simulink model "EEG_Acquire_P300_Train_B"  (R2015b)
settings: Solver=FixedStepDiscrete  StartTime=0.0  StopTime=6000  FixedStep=1/250  MaxStep=1/250  RelTol=1e-3
InitFcn:
  | clear global handle
  | 
  | clear global userData
undefined symbols (not defined in the file or in its folder): gcf
settings Model: Creator=ankit  LastModifiedBy=Sun Han
settings SolverCC: AutoInsertRateTranBlk=on  InsertRTBMode=Always
settings DataIOCC: LimitDataPoints=off  SaveFormat=Array  SignalLoggingSaveFormat=ModelDataLogs
settings OptimizationCC: ExpressionDepthLimit=2147483647  InitFltsAndDblsToZero=on
settings DebuggingCC: SaveWithParameterizedLinksMsg=none  UnderspecifiedInitializationDetection=Classic  MergeDetectMultiDrivingBlocksExec=none  SignalResolutionControl=TryResolveAllWithWarning  SolverPrmCheckMsg=warning  MultiTaskDSMMsg=warning  MultiTaskCondExecSysMsg=none  FcnCallInpInsideContextMsg=UseLocalSettings  StateNameClashWarn=warning
settings HardwareCC: ProdBitPerPointer=32  ProdLargestAtomicFloat=None  ProdIntDivRoundTo=Undefined  ProdEndianess=Unspecified  ProdWordSize=32  ProdHWDeviceType=32-bit Generic
settings GRTTargetCC: TargetFcnLib=ansi_tfl_tmw.mat  GeneratePreprocessorConditionals=Disable all  CombineOutputUpdateFcns=off  GRTInterface=on
settings ConfigComp: CovModelRefEnable=Off  CovSFcnEnable=off

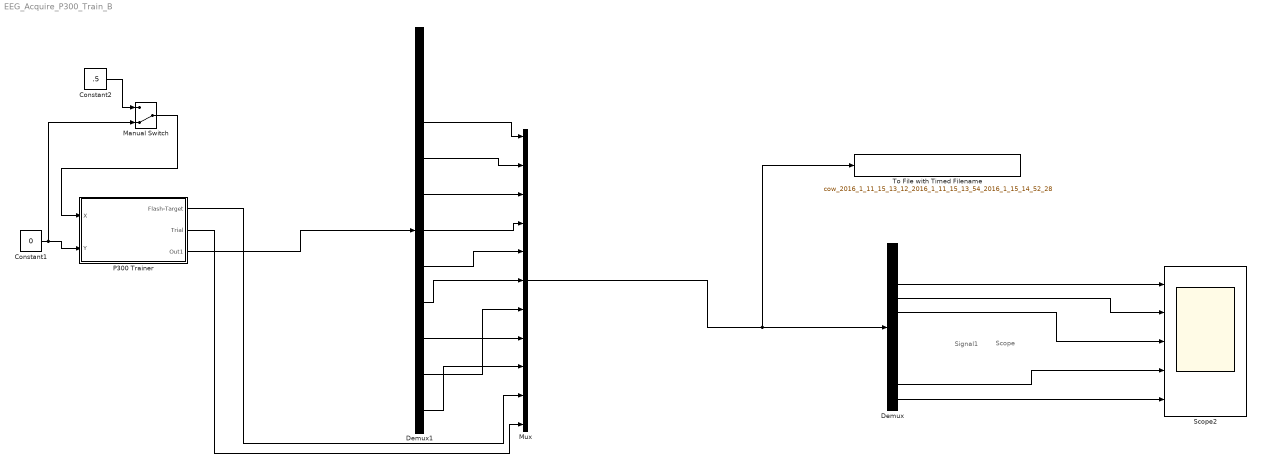
== system EEG_Acquire_P300_Train_B ==
  note: Scope
  note: Signal1
  Constant1 : Constant  Value=0
  Constant2 : Constant  Value=.5
  Demux : Demux  Outputs=11
  Demux1 : Demux  Outputs=11
  Manual Switch : ManualSwitch  CurrentSetting=0
  Mux : Mux  Inputs=11
  P300 Trainer : Subsystem  StopFcn=close(gcf)  mask(Single Character Flash Speller){flashtime=100, darktime=300, flashnum=3, imagescaling=0.75, centerout=0.3, cuescale=0.5, mode=Training, paramode=Pick 8, COMPort=COM12, SPS=250}
      mask prompts: flashtime "Flash time [ms]:"; darktime "Dark time [ms]:"; flashnum "Number of Flash(s)"; imagescaling "Target Scale"; centerout "Target Distance"; cuescale "Cue Scale"; paramode "Paradigm 4/8"; COMPort "COM Port"
      mask help: Displays a 36 character matrix. Each character is flashing up for a specific time in a random and sequential order. The dark time is the time between the characters.
      mask Help:
      | Displays a 36 character matrix. Each character is flashing up for a specific time in a random and sequential order. The dark time is the time between the characters. If the character is flashing up the ID-Flash is transmitted for the Signal Processing. Flash contains the ID of every character. Target is one if a specific character for the copy spelling mode flashes up. <br><br>
      | 
      | Mode - can be Copy Spelling or Free Spelling<br><br>
      | Flash time [ms] - time that character is shown on screen <br><br>
      | Dark time [ms] - time between the characters
      mask TypeOptions mode: Free Run | Training
      mask TypeOptions paramode: Pick 4 | Pick 8
      mask TypeOptions COMPort: COM1 | COM2 | COM3 | COM4 | COM5 | COM6 | COM7 | COM8 | COM9 | COM10 | COM11 | COM12 | COM13 | COM14 | COM15 | COM16 | COM17 | COM18 | COM19 | COM20
      mask TypeOptions SPS: 250 | 500 | 1000 | 2000 | 4000
      mask Display:
      | port_label('output',1,'Flash')
      | port_label('output',2,'Trial')
      | port_label('output',3,'EEGData')
      | port_label('input',1,'X')
      | port_label('input',2,'Y')
  Scope2 : Scope  NumInputPorts=5
  To File with Timed Filename : ToFile  InitFcn=|  StopFcn=|  Filename=cow_2016_1_11_15_13_12_2016_1_11_15_13_54_2016_1_15_14_52_28  MatrixName=y
      InitFcn=|
      | time=clock;                                                                                                                                                        
      | filenameToFilebase =  get_param(gcb,'Filename');                                                                                                                   
      | rename = [filenameToFilebase '_' num2str(time(1)) '_' num2str(time(2)) '_' num2str(time(3)) '_' num2str(time(4)) '_' num2str(time(5)) '_' num2str(round(time(6)))];
      | set_param(gcb,'Filename',rename);                                 clear time;                                                       clear rename;
      StopFcn=|
      | set_param(gcb,'Filename',filenameToFilebase);
      |                                              
      | clear filenameToFilebase
      settings: AttributesFormatString=Enter Base name, time will be added
  wires:
  Demux/5 -> Scope2/3
  Demux1/3 -> Mux/1
  Demux1/4 -> Mux/2
  Demux1/5 -> Mux/3
  Demux1/6 -> Mux/4
  Demux1/7 -> Mux/5
  Demux1/8 -> Mux/6
  Demux1/9 -> Mux/7
  Demux1/10 -> Mux/8
  Demux/3 -> Scope2/1
  Demux/4 -> Scope2/2
  Demux1/11 -> Mux/9
  P300 Trainer/3(Out1) -> Demux1/1
  P300 Trainer/1(Flash-Target) -> Mux/10
  P300 Trainer/2(Trial) -> Mux/11
  Mux/1 -> To File with Timed Filename/1, Demux/1
  Demux/11 -> Scope2/5
  Demux/10 -> Scope2/4
  Constant1/1 -> Manual Switch/2, P300 Trainer/2(Y)
  Manual Switch/1 -> P300 Trainer/1(X)
  Constant2/1 -> Manual Switch/1

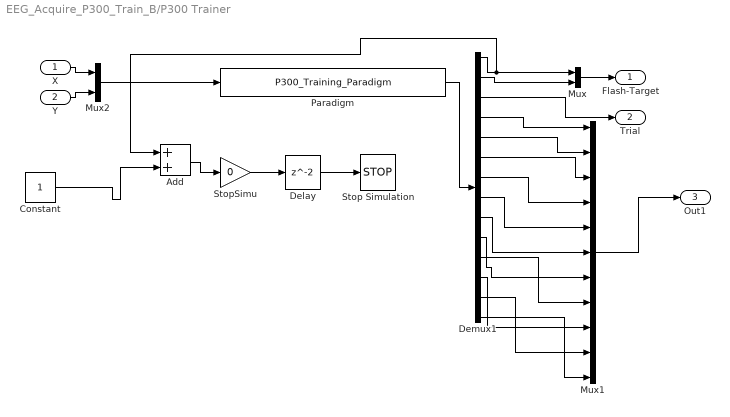
== system EEG_Acquire_P300_Train_B/P300 Trainer ==
  X : Inport
  Y : Inport  Port=2
  Add : Sum
  Constant : Constant
  Delay : Delay
  Demux1 : Demux  Outputs=14
  Mux : Mux  Inputs=2
  Mux1 : Mux  Inputs=11
  Mux2 : Mux  Inputs=2
  Paradigm : S-Function  FunctionName=P300_Training_Paradigm  Parameters=flashtime,darktime,mode,flashnum,paramode,imagescaling,centerout,cuescale,COMPort,SPS  SFunctionDeploymentMode=off  EnableBusSupport=off
  Stop Simulation : Stop
  StopSimu : Gain  Gain=0
  Flash-Target : Outport
  Trial : Outport  Port=2
  Out1 : Outport  Port=3
  wires:
  Paradigm/1 -> Demux1/1
  Constant/1 -> Add/2
  StopSimu/1 -> Delay/1
  Demux1/1 -> Add/1, Mux/1
  Demux1/2 -> Mux/2
  Mux/1 -> Flash-Target/1
  Demux1/3 -> Trial/1
  Demux1/4 -> Mux1/1
  Demux1/5 -> Mux1/2
  Demux1/6 -> Mux1/3
  Demux1/7 -> Mux1/4
  Demux1/8 -> Mux1/5
  Demux1/9 -> Mux1/6
  Demux1/10 -> Mux1/7
  Demux1/11 -> Mux1/8
  Demux1/12 -> Mux1/9
  Demux1/13 -> Mux1/10
  Demux1/14 -> Mux1/11
  Mux1/1 -> Out1/1
  X/1 -> Mux2/1
  Y/1 -> Mux2/2
  Mux2/1 -> Paradigm/1
  Delay/1 -> Stop Simulation/1
  Add/1 -> StopSimu/1
